simulink model "pattern_separation"  (R2019b)
settings: Solver=FixedStepAuto  StartTime=1  StopTime=simulationtime  FixedStep=stepsize  RelTol=1e-3
values from neighbouring files (symbols this model uses):
  a1 = 0.02    [simulation.m]
  a2 = 0.02    [simulation.m]
  b1 = 0.025    [simulation.m]
  b2 = 0.04    [simulation.m]
  c1 = -65    [simulation.m]
  C1 = normrnd(100,10,[1,nrofgranulecells])    [simulation.m]
  c2 = -65    [simulation.m]
  C2 = normrnd(100,10,[1,nrofinterneurons])    [simulation.m]
  d1 = 6    [simulation.m]
  d2 = 2    [simulation.m]
  inputset = inputsets{no_input}    [simulation.m]
  k1 = 0.25    [simulation.m]
  k2 = 0.25    [simulation.m]
  minimum_saturation_limit_1 = -80    [simulation.m]
  minimum_saturation_limit_2 = -100    [simulation.m]
  noumberofevents = 500    [simulation.m]
  Re = 230    [simulation.m]
  simulationtime = 2000    [simulation.m]
  stepsize = 1    [simulation.m]
  ve1 = -5    [simulation.m]
  ve2 = -80    [simulation.m]
  vr1 = -60    [simulation.m]
  vr2 = -65    [simulation.m]
  vt1 = -55    [simulation.m]
  vt2 = -48    [simulation.m]
undefined symbols (not defined in the file or in its folder): conductancemaxima1, conductancemaxima2, conductancemaxima3, decaytimes1, decaytimes2, decaytimes3, DiscIntNeverNeededParam, Nd, trace
(part 1 of 5)
settings Model: Creator=agorlewicz  LastModifiedBy=agorlewicz
settings OptimizationCC: BlockReduction=off  DefaultParameterBehavior=Inlined  BufferReuse=off

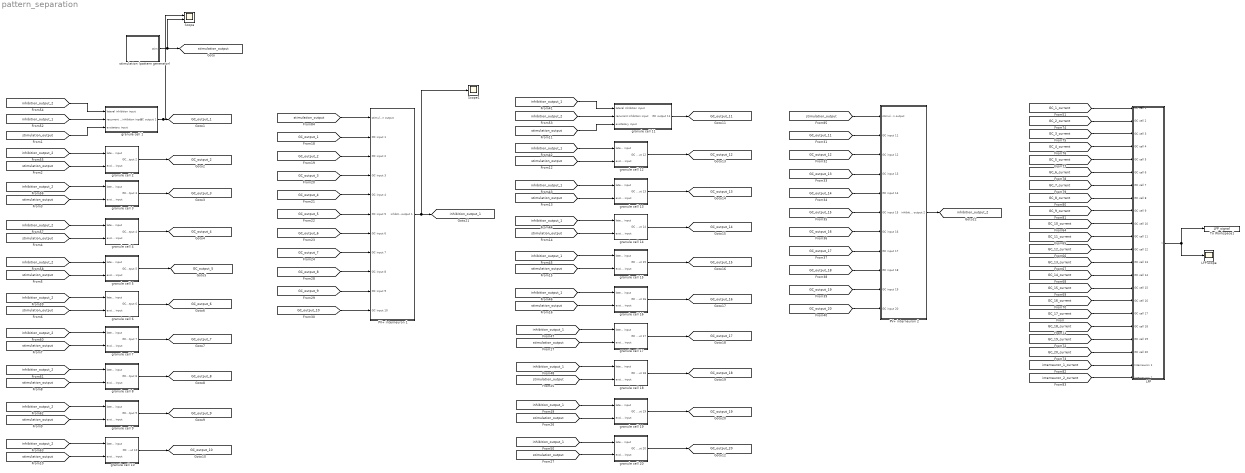
== system pattern_separation ==
  LFP : Subsystem
  LFP scope : Scope
  PV+ interneuron 1 : Subsystem
  PV+ interneuron 2 : Subsystem
  Scope : Scope  NumInputPorts=2
  Scope1 : Scope
  To Workspace1 : ToWorkspace  VariableName=LFP_signal  SampleTime=-1
  granule cell 1 : Subsystem
  granule cell 10 : Subsystem
  granule cell 11 : Subsystem
  granule cell 12 : Subsystem
  granule cell 13 : Subsystem
  granule cell 14 : Subsystem
  granule cell 15 : Subsystem
  granule cell 16 : Subsystem
  granule cell 17 : Subsystem
  granule cell 18 : Subsystem
  granule cell 19 : Subsystem
  granule cell 2 : Subsystem
  granule cell 20 : Subsystem
  granule cell 3 : Subsystem
  granule cell 4 : Subsystem
  granule cell 5 : Subsystem
  granule cell 6 : Subsystem
  granule cell 7 : Subsystem
  granule cell 8 : Subsystem
  granule cell 9 : Subsystem
  stimulation (pattern generator) : Subsystem
  tag scope: GC_output_10=global, GC_output_11=global, GC_output_12=global, GC_output_13=global, GC_output_14=global, GC_output_15=global, GC_output_16=global, GC_output_17=global, GC_output_18=global, GC_output_19=global, GC_output_1=global, GC_output_20=global, GC_output_2=global, GC_output_3=global, GC_output_4=global, GC_output_5=global, GC_output_6=global, GC_output_7=global, GC_output_8=global, GC_output_9=global, inhibition_output_1=global, inhibition_output_2=global, stimulation_output=global
  wires:
  stimulation (pattern generator)/1(stim) -> Scope/2, [stimulation_output]
  [stimulation_output] -> granule cell 1/3(excitatory input)
  [stimulation_output] -> granule cell 2/2(excitatory input)
  [stimulation_output] -> granule cell 3/2(excitatory input)
  [stimulation_output] -> granule cell 4/2(excitatory input)
  [stimulation_output] -> granule cell 5/2(excitatory input)
  [stimulation_output] -> granule cell 8/2(excitatory input)
  [stimulation_output] -> granule cell 7/2(excitatory input)
  [stimulation_output] -> granule cell 6/2(excitatory input)
  [stimulation_output] -> granule cell 9/2(excitatory input)
  [stimulation_output] -> granule cell 10/2(excitatory input)
  [stimulation_output] -> granule cell 11/3(excitatory input)
  [stimulation_output] -> granule cell 12/2(excitatory input)
  [stimulation_output] -> granule cell 13/2(excitatory input)
  [stimulation_output] -> granule cell 14/2(excitatory input)
  [stimulation_output] -> granule cell 15/2(excitatory input)
  [stimulation_output] -> granule cell 16/2(excitatory input)
  [stimulation_output] -> granule cell 18/2(excitatory input)
  [stimulation_output] -> granule cell 19/2(excitatory input)
  [stimulation_output] -> granule cell 17/2(excitatory input)
  [stimulation_output] -> granule cell 20/2(excitatory input)
  granule cell 1/1(GC output 1) -> Scope/1, [GC_output_1]
  [GC_output_1] -> PV+ interneuron 1/2(" GC input 1")
  granule cell 2/1(GC output 2) -> [GC_output_2]
  [GC_output_2] -> PV+ interneuron 1/3(" GC input 2")
  granule cell 3/1(GC output 3) -> [GC_output_3]
  [GC_output_3] -> PV+ interneuron 1/4(" GC input 3")
  granule cell 4/1(GC output 4) -> [GC_output_4]
  granule cell 5/1(GC output 5) -> [GC_output_5]
  granule cell 6/1(GC output 6) -> [GC_output_6]
  granule cell 7/1(GC output 7) -> [GC_output_7]
  granule cell 8/1(GC output 8) -> [GC_output_8]
  granule cell 9/1(GC output 9) -> [GC_output_9]
  granule cell 10/1(GC output 10) -> [GC_output_10]
  [GC_output_4] -> PV+ interneuron 1/5(" GC input 4")
  [GC_output_5] -> PV+ interneuron 1/6(" GC input 5")
  [GC_output_6] -> PV+ interneuron 1/7(" GC input 6")
  [GC_output_7] -> PV+ interneuron 1/8(" GC input 7")
  [GC_output_8] -> PV+ interneuron 1/9(" GC input 8")
  [GC_output_9] -> PV+ interneuron 1/10(GC input 9)
  [GC_output_10] -> PV+ interneuron 1/11(GC input 10)
  granule cell 11/1(GC output 11) -> [GC_output_11]
  granule cell 12/1(GC output 12) -> [GC_output_12]
  granule cell 13/1(GC output 13) -> [GC_output_13]
  granule cell 14/1(GC output 14) -> [GC_output_14]
  granule cell 15/1(GC output 15) -> [GC_output_15]
  granule cell 16/1(GC output 16) -> [GC_output_16]
  granule cell 17/1(GC output 17) -> [GC_output_17]
  granule cell 18/1(GC output 18) -> [GC_output_18]
  granule cell 19/1(GC output 19) -> [GC_output_19]
  granule cell 20/1(GC output 20) -> [GC_output_20]
  [GC_output_11] -> PV+ interneuron 2/2(" GC input 11")
  [GC_output_12] -> PV+ interneuron 2/3(" GC input 12")
  [GC_output_13] -> PV+ interneuron 2/4(" GC input 13")
  [GC_output_14] -> PV+ interneuron 2/5(" GC input 14")
  [GC_output_15] -> PV+ interneuron 2/6(" GC input 15")
  [GC_output_16] -> PV+ interneuron 2/7(" GC input 16")
  [GC_output_17] -> PV+ interneuron 2/8(" GC input 17")
  [GC_output_18] -> PV+ interneuron 2/9(" GC input 18")
  [GC_output_19] -> PV+ interneuron 2/10(GC input 19)
  [GC_output_20] -> PV+ interneuron 2/11(GC input 20)
  PV+ interneuron 1/1(inhibition output 1) -> [inhibition_output_1], Scope1/1
  [inhibition_output_1] -> granule cell 11/1(lateral inhibition input)
  [inhibition_output_1] -> granule cell 12/1(lateral inhibition input)
  [inhibition_output_1] -> granule cell 13/1(lateral inhibition input)
  [inhibition_output_1] -> granule cell 14/1(lateral inhibition input)
  [inhibition_output_1] -> granule cell 15/1(lateral inhibition input)
  [inhibition_output_1] -> granule cell 16/1(lateral inhibition input)
  [inhibition_output_1] -> granule cell 17/1(lateral inhibition input)
  [inhibition_output_1] -> granule cell 18/1(lateral inhibition input)
  [inhibition_output_1] -> granule cell 19/1(lateral inhibition input)
  [inhibition_output_1] -> granule cell 20/1(lateral inhibition input)
  [inhibition_output_1] -> granule cell 1/2(recurrent inhibition input)
  PV+ interneuron 2/1(inhibition output 2) -> [inhibition_output_2]
  [inhibition_output_2] -> granule cell 11/2(recurrent inhibition input)
  [inhibition_output_2] -> granule cell 1/1(lateral inhibition input)
  [inhibition_output_2] -> granule cell 2/1(lateral inhibition input)
  [inhibition_output_2] -> granule cell 3/1(lateral inhibition input)
  [inhibition_output_2] -> granule cell 4/1(lateral inhibition input)
  [inhibition_output_2] -> granule cell 5/1(lateral inhibition input)
  [inhibition_output_2] -> granule cell 6/1(lateral inhibition input)
  [inhibition_output_2] -> granule cell 7/1(lateral inhibition input)
  [inhibition_output_2] -> granule cell 8/1(lateral inhibition input)
  [inhibition_output_2] -> granule cell 9/1(lateral inhibition input)
  [inhibition_output_2] -> granule cell 10/1(lateral inhibition input)
  [GC_11_current] -> LFP/11(GC cell 11)
  [GC_9_current] -> LFP/9(GC cell 9)
  [GC_12_current] -> LFP/12(GC cell 12)
  [GC_14_current] -> LFP/14(GC cell 14)
  [GC_1_current] -> LFP/1("GC cell 1 ")
  [GC_13_current] -> LFP/13(GC cell 13)
  [GC_16_current] -> LFP/16(GC cell 16)
  [GC_17_current] -> LFP/17(GC cell 17)
  [GC_4_current] -> LFP/4("GC cell 4 ")
  [GC_5_current] -> LFP/5(GC cell 5)
  [GC_18_current] -> LFP/18(GC cell 18)
  [GC_8_current] -> LFP/8("GC cell 8 ")
  [GC_6_current] -> LFP/6(GC cell 6)
  [GC_7_current] -> LFP/7(GC cell 7)
  LFP/1(v) -> To Workspace1/1, LFP scope/1
  [GC_15_current] -> LFP/15(GC cell 15)
  [GC_3_current] -> LFP/3("GC cell 3 ")
  [GC_10_current] -> LFP/10(GC cell 10)
  [GC_19_current] -> LFP/19(GC cell 19)
  [GC_2_current] -> LFP/2("GC cell 2 ")
  [GC_20_current] -> LFP/20(GC cell 20)
  [interneuron_1_current] -> LFP/21(Interneuron 1)
  [interneuron_2_current] -> LFP/22(Interneuron 2)
  [stimulation_output] -> PV+ interneuron 1/1(stimulation output)
  [stimulation_output] -> PV+ interneuron 2/1(stimulation output)

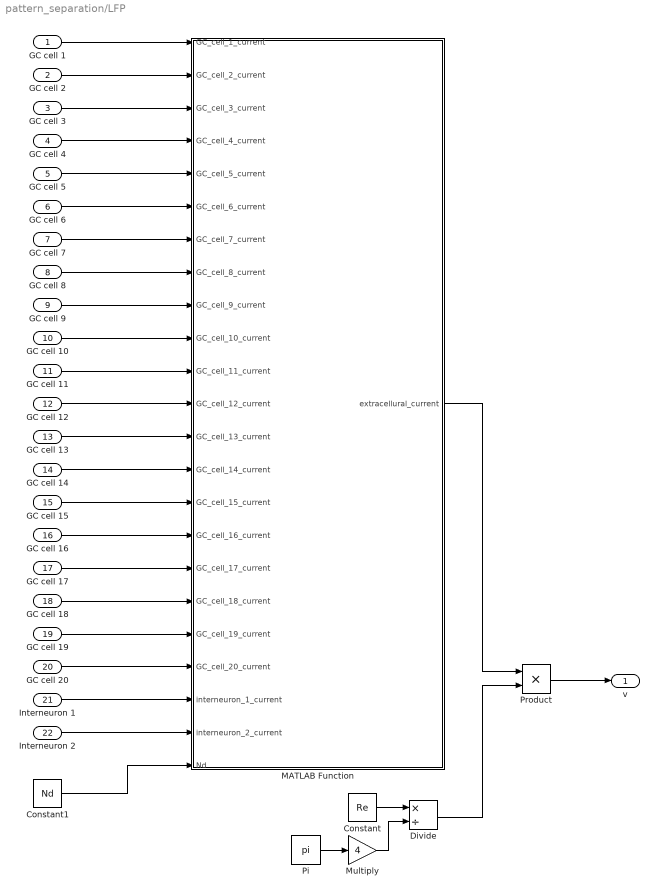
== system pattern_separation/LFP ==
  "GC cell 1 " : Inport
  "GC cell 2 " : Inport  Port=2
  "GC cell 3 " : Inport  Port=3
  "GC cell 4 " : Inport  Port=4
  GC cell 5 : Inport  Port=5
  GC cell 6 : Inport  Port=6
  GC cell 7 : Inport  Port=7
  "GC cell 8 " : Inport  Port=8
  GC cell 9 : Inport  Port=9
  GC cell 10 : Inport  Port=10
  GC cell 11 : Inport  Port=11
  GC cell 12 : Inport  Port=12
  GC cell 13 : Inport  Port=13
  GC cell 14 : Inport  Port=14
  GC cell 15 : Inport  Port=15
  GC cell 16 : Inport  Port=16
  GC cell 17 : Inport  Port=17
  GC cell 18 : Inport  Port=18
  GC cell 19 : Inport  Port=19
  GC cell 20 : Inport  Port=20
  Interneuron 1 : Inport  Port=21
  Interneuron 2 : Inport  Port=22
  Constant : Constant  Value=Re
  Constant1 : Constant  Value=Nd
  Divide : Product  Inputs=*/
  MATLAB Function : MATLAB Function  TreatAsAtomicUnit=on
  Multiply : Gain  Gain=4
  Pi : Constant  Value=pi  OutDataTypeStr=Inherit: Inherit via back propagation
  Product : Product
  v : Outport
  wires:
  Constant/1 -> Divide/1
  Pi/1 -> Multiply/1
  Multiply/1 -> Divide/2
  Constant1/1 -> MATLAB Function/23(Nd)
  MATLAB Function/1(extracellural_current) -> Product/1
  Divide/1 -> Product/2
  Product/1 -> v/1
  GC cell 20/1 -> MATLAB Function/20(GC_cell_20_current)
  GC cell 19/1 -> MATLAB Function/19(GC_cell_19_current)
  GC cell 18/1 -> MATLAB Function/18(GC_cell_18_current)
  GC cell 17/1 -> MATLAB Function/17(GC_cell_17_current)
  GC cell 16/1 -> MATLAB Function/16(GC_cell_16_current)
  GC cell 15/1 -> MATLAB Function/15(GC_cell_15_current)
  GC cell 14/1 -> MATLAB Function/14(GC_cell_14_current)
  GC cell 13/1 -> MATLAB Function/13(GC_cell_13_current)
  GC cell 12/1 -> MATLAB Function/12(GC_cell_12_current)
  GC cell 11/1 -> MATLAB Function/11(GC_cell_11_current)
  GC cell 10/1 -> MATLAB Function/10(GC_cell_10_current)
  GC cell 9/1 -> MATLAB Function/9(GC_cell_9_current)
  "GC cell 8 "/1 -> MATLAB Function/8(GC_cell_8_current)
  "GC cell 1 "/1 -> MATLAB Function/1(GC_cell_1_current)
  "GC cell 2 "/1 -> MATLAB Function/2(GC_cell_2_current)
  "GC cell 3 "/1 -> MATLAB Function/3(GC_cell_3_current)
  "GC cell 4 "/1 -> MATLAB Function/4(GC_cell_4_current)
  GC cell 5/1 -> MATLAB Function/5(GC_cell_5_current)
  GC cell 6/1 -> MATLAB Function/6(GC_cell_6_current)
  GC cell 7/1 -> MATLAB Function/7(GC_cell_7_current)
  Interneuron 1/1 -> MATLAB Function/21(interneuron_1_current)
  Interneuron 2/1 -> MATLAB Function/22(interneuron_2_current)

== system pattern_separation/PV+ interneuron 1 ==
  stimulation output : Inport
  " GC input 1" : Inport  Port=2
  " GC input 2" : Inport  Port=3
  " GC input 3" : Inport  Port=4
  " GC input 4" : Inport  Port=5
  " GC input 5" : Inport  Port=6
  " GC input 6" : Inport  Port=7
  " GC input 7" : Inport  Port=8
  " GC input 8" : Inport  Port=9
  GC input 9 : Inport  Port=10
  GC input 10 : Inport  Port=11
  Add2 : Sum  Inputs=+++++++++++
  Constant3 : Constant  SampleTime=-1
  Constant4 : Constant  Value=decaytimes3  SampleTime=-1
  Constant5 : Constant  Value=conductancemaxima3  SampleTime=-1
  Constant7 : Constant  Value=0  SampleTime=-1
  Data Type Conversion1 : DataTypeConversion  OutDataTypeStr=double
  Discrete-Time Integrator1 : DiscreteIntegrator  gainval=1/stepsize  ExternalReset=sampled level  SampleTime=-1  ICPrevOutput=DiscIntNeverNeededParam  ICPrevScaledInput=DiscIntNeverNeededParam
  Floor1 : Rounding
  Integrator1 : Integrator  ExternalReset=level hold
  MATLAB Function1 : MATLAB Function  TreatAsAtomicUnit=on
  Memory1 : Memory  InheritSampleTime=on
  Product2 : Product
  Relational Operator1 : RelationalOperator  Operator=>  OutDataTypeStr=boolean  RndMeth=Simplest
  Uniform Random Number1 : UniformRandomNumber  Minimum=1  Maximum=noumberofevents  Seed=41  SampleTime=stepsize
  interneuron : Subsystem
  single exp EPSCs generator (ff synapse) : Subsystem
  inhibition output 1 : Outport
  tag scope: interneuron_1_current=global
  wires:
  interneuron/1(output) -> inhibition output 1/1
  Memory1/1 -> Product2/1, Discrete-Time Integrator1/2, Integrator1/2
  Uniform Random Number1/1 -> Floor1/1
  Constant4/1 -> MATLAB Function1/2(decaytimes3)
  Floor1/1 -> Product2/2
  Constant5/1 -> MATLAB Function1/3(conductancemaxima3)
  Integrator1/1 -> single exp EPSCs generator (ff synapse)/1(event time)
  MATLAB Function1/1(decaytime) -> single exp EPSCs generator (ff synapse)/2(decay time constant)
  MATLAB Function1/2(conductancemaximum) -> single exp EPSCs generator (ff synapse)/3(conductance maximum)
  Constant3/1 -> Integrator1/1
  Product2/1 -> Discrete-Time Integrator1/1
  Discrete-Time Integrator1/1 -> MATLAB Function1/1(eventnoumber)
  single exp EPSCs generator (ff synapse)/1(postsynaptic current) -> [interneuron_1_current], interneuron/1(postsynaptic current)
  Constant7/1 -> Relational Operator1/2
  Relational Operator1/1 -> Data Type Conversion1/1
  " GC input 1"/1 -> Add2/2
  " GC input 2"/1 -> Add2/3
  Add2/1 -> Relational Operator1/1
  Data Type Conversion1/1 -> Memory1/1
  " GC input 3"/1 -> Add2/4
  " GC input 4"/1 -> Add2/5
  " GC input 5"/1 -> Add2/6
  " GC input 6"/1 -> Add2/7
  " GC input 7"/1 -> Add2/8
  " GC input 8"/1 -> Add2/9
  GC input 9/1 -> Add2/10
  GC input 10/1 -> Add2/11
  stimulation output/1 -> Add2/1

== system pattern_separation/PV+ interneuron 2 ==
  stimulation output : Inport
  " GC input 11" : Inport  Port=2
  " GC input 12" : Inport  Port=3
  " GC input 13" : Inport  Port=4
  " GC input 14" : Inport  Port=5
  " GC input 15" : Inport  Port=6
  " GC input 16" : Inport  Port=7
  " GC input 17" : Inport  Port=8
  " GC input 18" : Inport  Port=9
  GC input 19 : Inport  Port=10
  GC input 20 : Inport  Port=11
  Add2 : Sum  Inputs=+++++++++++
  Constant3 : Constant  SampleTime=-1
  Constant4 : Constant  Value=decaytimes3  SampleTime=-1
  Constant5 : Constant  Value=conductancemaxima3  SampleTime=-1
  Constant7 : Constant  Value=0  SampleTime=-1
  Data Type Conversion1 : DataTypeConversion  OutDataTypeStr=double
  Discrete-Time Integrator1 : DiscreteIntegrator  gainval=1/stepsize  ExternalReset=sampled level  SampleTime=-1  ICPrevOutput=DiscIntNeverNeededParam  ICPrevScaledInput=DiscIntNeverNeededParam
  Floor1 : Rounding
  Integrator1 : Integrator  ExternalReset=level hold
  MATLAB Function1 : MATLAB Function  TreatAsAtomicUnit=on
  Memory1 : Memory  InheritSampleTime=on
  Product2 : Product
  Relational Operator1 : RelationalOperator  Operator=>  OutDataTypeStr=boolean  RndMeth=Simplest
  Uniform Random Number1 : UniformRandomNumber  Minimum=1  Maximum=noumberofevents  Seed=42  SampleTime=stepsize
  interneuron : Subsystem
  single exp EPSCs generator (ff synapse) : Subsystem
  inhibition output 2 : Outport
  tag scope: interneuron_2_current=global
  wires:
  interneuron/1(output) -> inhibition output 2/1
  Memory1/1 -> Product2/1, Discrete-Time Integrator1/2, Integrator1/2
  Uniform Random Number1/1 -> Floor1/1
  Constant4/1 -> MATLAB Function1/2(decaytimes3)
  Floor1/1 -> Product2/2
  Constant5/1 -> MATLAB Function1/3(conductancemaxima3)
  Integrator1/1 -> single exp EPSCs generator (ff synapse)/1(event time)
  MATLAB Function1/1(decaytime) -> single exp EPSCs generator (ff synapse)/2(decay time constant)
  MATLAB Function1/2(conductancemaximum) -> single exp EPSCs generator (ff synapse)/3(conductance maximum)
  Constant3/1 -> Integrator1/1
  Product2/1 -> Discrete-Time Integrator1/1
  Discrete-Time Integrator1/1 -> MATLAB Function1/1(eventnoumber)
  single exp EPSCs generator (ff synapse)/1(postsynaptic current) -> [interneuron_2_current], interneuron/1(postsynaptic current)
  Constant7/1 -> Relational Operator1/2
  Relational Operator1/1 -> Data Type Conversion1/1
  " GC input 11"/1 -> Add2/2
  " GC input 12"/1 -> Add2/3
  Add2/1 -> Relational Operator1/1
  Data Type Conversion1/1 -> Memory1/1
  " GC input 13"/1 -> Add2/4
  " GC input 14"/1 -> Add2/5
  " GC input 15"/1 -> Add2/6
  " GC input 16"/1 -> Add2/7
  " GC input 17"/1 -> Add2/8
  " GC input 18"/1 -> Add2/9
  GC input 19/1 -> Add2/10
  GC input 20/1 -> Add2/11
  stimulation output/1 -> Add2/1

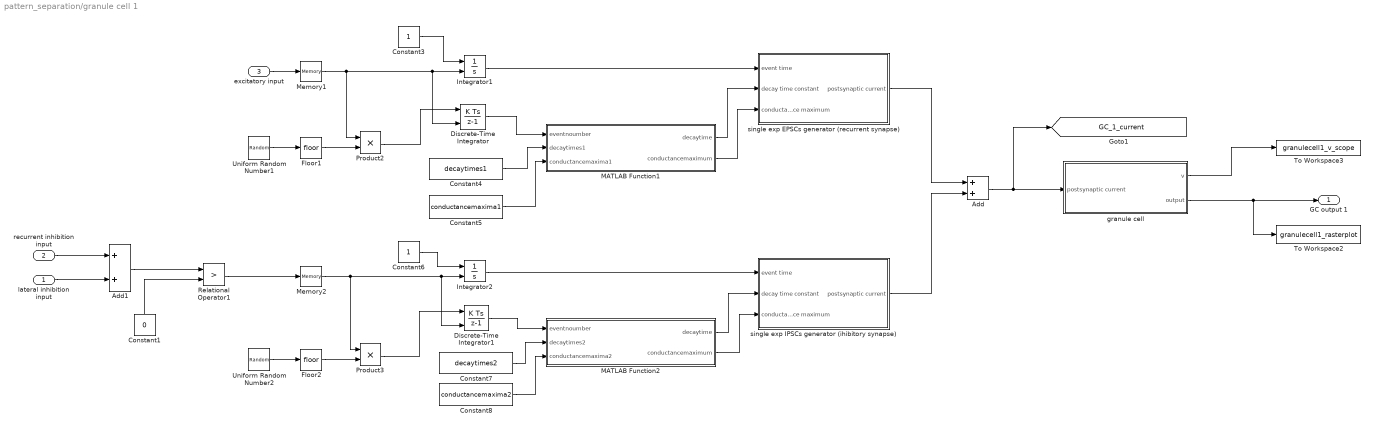
== system pattern_separation/granule cell 1 ==
  lateral inhibition input : Inport
  recurrent inhibition input : Inport  Port=2
  excitatory input : Inport  Port=3
  Add : Sum
  Add1 : Sum
  Constant1 : Constant  Value=0  SampleTime=-1
  Constant3 : Constant  SampleTime=-1
  Constant4 : Constant  Value=decaytimes1  SampleTime=-1
  Constant5 : Constant  Value=conductancemaxima1  SampleTime=-1
  Constant6 : Constant  SampleTime=-1
  Constant7 : Constant  Value=decaytimes2  SampleTime=-1
  Constant8 : Constant  Value=conductancemaxima2  SampleTime=-1
  Discrete-Time Integrator : DiscreteIntegrator  gainval=1/stepsize  ExternalReset=sampled level  SampleTime=-1  ICPrevOutput=DiscIntNeverNeededParam  ICPrevScaledInput=DiscIntNeverNeededParam
  Discrete-Time Integrator1 : DiscreteIntegrator  gainval=1/stepsize  ExternalReset=sampled level  SampleTime=-1  ICPrevOutput=DiscIntNeverNeededParam  ICPrevScaledInput=DiscIntNeverNeededParam
  Floor1 : Rounding
  Floor2 : Rounding
  Integrator1 : Integrator  ExternalReset=level hold
  Integrator2 : Integrator  ExternalReset=level hold
  MATLAB Function1 : MATLAB Function  TreatAsAtomicUnit=on
  MATLAB Function2 : MATLAB Function  TreatAsAtomicUnit=on
  Memory1 : Memory  InheritSampleTime=on
  Memory2 : Memory  InheritSampleTime=on
  Product2 : Product
  Product3 : Product
  Relational Operator1 : RelationalOperator  Operator=>  OutDataTypeStr=boolean  RndMeth=Simplest
  To Workspace2 : ToWorkspace  VariableName=granulecell1_rasterplot  SampleTime=-1
  To Workspace3 : ToWorkspace  VariableName=granulecell1_v_scope  SampleTime=-1
  Uniform Random Number1 : UniformRandomNumber  Minimum=1  Maximum=noumberofevents  Seed=1  SampleTime=stepsize
  Uniform Random Number2 : UniformRandomNumber  Minimum=1  Maximum=noumberofevents  Seed=2  SampleTime=stepsize
  granule cell : Subsystem
  single exp EPSCs generator (recurrent synapse) : Subsystem
  single exp IPSCs generator (ihibitory synapse) : Subsystem
  GC output 1 : Outport
  tag scope: GC_1_current=global
  wires:
  Discrete-Time Integrator/1 -> MATLAB Function1/1(eventnoumber)
  Memory1/1 -> Product2/1, Discrete-Time Integrator/2, Integrator1/2
  granule cell/2(output) -> To Workspace2/1, GC output 1/1
  MATLAB Function2/2(conductancemaximum) -> single exp IPSCs generator (ihibitory synapse)/3(conductance maximum)
  Uniform Random Number1/1 -> Floor1/1
  Uniform Random Number2/1 -> Floor2/1
  excitatory input/1 -> Memory1/1
  single exp EPSCs generator (recurrent synapse)/1(postsynaptic current) -> Add/1
  Product3/1 -> Discrete-Time Integrator1/1
  Floor1/1 -> Product2/2
  Constant3/1 -> Integrator1/1
  single exp IPSCs generator (ihibitory synapse)/1(postsynaptic current) -> Add/2
  Product2/1 -> Discrete-Time Integrator/1
  granule cell/1(v) -> To Workspace3/1
  MATLAB Function1/1(decaytime) -> single exp EPSCs generator (recurrent synapse)/2(decay time constant)
  MATLAB Function2/1(decaytime) -> single exp IPSCs generator (ihibitory synapse)/2(decay time constant)
  Integrator1/1 -> single exp EPSCs generator (recurrent synapse)/1(event time)
  Constant5/1 -> MATLAB Function1/3(conductancemaxima1)
  Memory2/1 -> Product3/1, Discrete-Time Integrator1/2, Integrator2/2
  MATLAB Function1/2(conductancemaximum) -> single exp EPSCs generator (recurrent synapse)/3(conductance maximum)
  Constant6/1 -> Integrator2/1
  Constant4/1 -> MATLAB Function1/2(decaytimes1)
  Constant7/1 -> MATLAB Function2/2(decaytimes2)
  Constant8/1 -> MATLAB Function2/3(conductancemaxima2)
  Floor2/1 -> Product3/2
  Integrator2/1 -> single exp IPSCs generator (ihibitory synapse)/1(event time)
  Discrete-Time Integrator1/1 -> MATLAB Function2/1(eventnoumber)
  Add1/1 -> Relational Operator1/1
  Constant1/1 -> Relational Operator1/2
  recurrent inhibition input/1 -> Add1/1
  lateral inhibition input/1 -> Add1/2
  Relational Operator1/1 -> Memory2/1
  Add/1 -> granule cell/1(postsynaptic current), [GC_1_current]

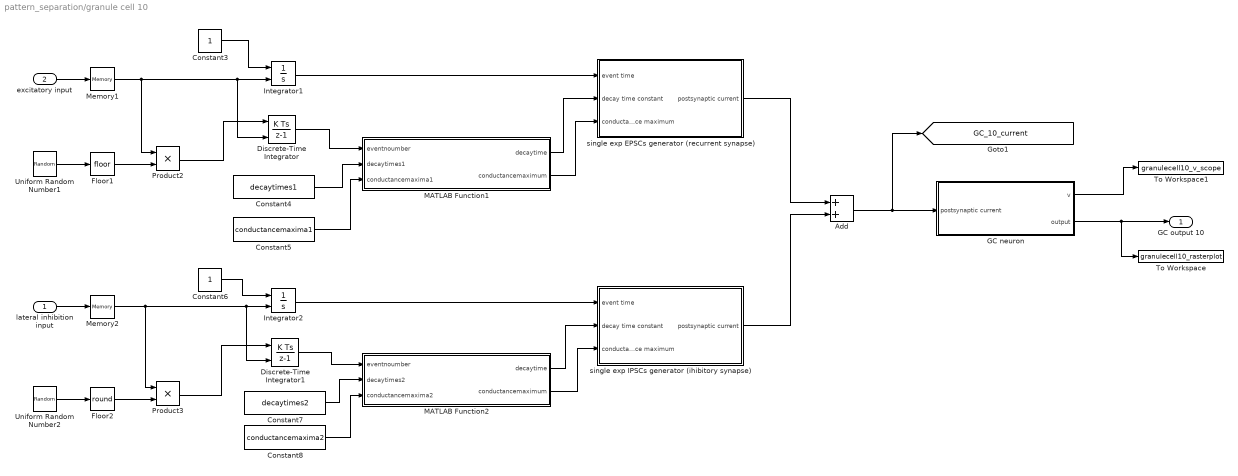
== system pattern_separation/granule cell 10 ==
  lateral inhibition input : Inport
  excitatory input : Inport  Port=2
  Add : Sum
  Constant3 : Constant  SampleTime=-1
  Constant4 : Constant  Value=decaytimes1  SampleTime=-1
  Constant5 : Constant  Value=conductancemaxima1  SampleTime=-1
  Constant6 : Constant  SampleTime=-1
  Constant7 : Constant  Value=decaytimes2  SampleTime=-1
  Constant8 : Constant  Value=conductancemaxima2  VectorParams1D=off  SampleTime=-1
  Discrete-Time Integrator : DiscreteIntegrator  gainval=1/stepsize  ExternalReset=sampled level  SampleTime=-1  ICPrevOutput=DiscIntNeverNeededParam  ICPrevScaledInput=DiscIntNeverNeededParam
  Discrete-Time Integrator1 : DiscreteIntegrator  gainval=1/stepsize  ExternalReset=sampled level  SampleTime=-1  ICPrevOutput=DiscIntNeverNeededParam  ICPrevScaledInput=DiscIntNeverNeededParam
  Floor1 : Rounding
  Floor2 : Rounding  Operator=round
  GC neuron : Subsystem
  Integrator1 : Integrator  ExternalReset=level hold
  Integrator2 : Integrator  ExternalReset=level hold
  MATLAB Function1 : MATLAB Function  TreatAsAtomicUnit=on
  MATLAB Function2 : MATLAB Function  TreatAsAtomicUnit=on
  Memory1 : Memory  InheritSampleTime=on
  Memory2 : Memory  InheritSampleTime=on
  Product2 : Product
  Product3 : Product
  To Workspace : ToWorkspace  VariableName=granulecell10_rasterplot  SampleTime=-1
  To Workspace1 : ToWorkspace  VariableName=granulecell10_v_scope  SampleTime=-1
  Uniform Random Number1 : UniformRandomNumber  Minimum=1  Maximum=noumberofevents  Seed=19  SampleTime=stepsize
  Uniform Random Number2 : UniformRandomNumber  Minimum=1  Maximum=noumberofevents  Seed=20  SampleTime=stepsize
  single exp EPSCs generator (recurrent synapse) : Subsystem
  single exp IPSCs generator (ihibitory synapse) : Subsystem
  GC output 10 : Outport
  tag scope: GC_10_current=global
  wires:
  GC neuron/1(v) -> To Workspace1/1
  GC neuron/2(output) -> To Workspace/1, GC output 10/1
  Constant7/1 -> MATLAB Function2/2(decaytimes2)
  Constant8/1 -> MATLAB Function2/3(conductancemaxima2)
  Discrete-Time Integrator1/1 -> MATLAB Function2/1(eventnoumber)
  Floor2/1 -> Product3/2
  Discrete-Time Integrator/1 -> MATLAB Function1/1(eventnoumber)
  MATLAB Function2/1(decaytime) -> single exp IPSCs generator (ihibitory synapse)/2(decay time constant)
  Product2/1 -> Discrete-Time Integrator/1
  Integrator2/1 -> single exp IPSCs generator (ihibitory synapse)/1(event time)
  Add/1 -> [GC_10_current], GC neuron/1(postsynaptic current)
  Memory2/1 -> Product3/1, Discrete-Time Integrator1/2, Integrator2/2
  single exp IPSCs generator (ihibitory synapse)/1(postsynaptic current) -> Add/2
  MATLAB Function1/1(decaytime) -> single exp EPSCs generator (recurrent synapse)/2(decay time constant)
  MATLAB Function1/2(conductancemaximum) -> single exp EPSCs generator (recurrent synapse)/3(conductance maximum)
  Constant6/1 -> Integrator2/1
  Constant4/1 -> MATLAB Function1/2(decaytimes1)
  Constant5/1 -> MATLAB Function1/3(conductancemaxima1)
  Integrator1/1 -> single exp EPSCs generator (recurrent synapse)/1(event time)
  Product3/1 -> Discrete-Time Integrator1/1
  single exp EPSCs generator (recurrent synapse)/1(postsynaptic current) -> Add/1
  lateral inhibition input/1 -> Memory2/1
  Floor1/1 -> Product2/2
  MATLAB Function2/2(conductancemaximum) -> single exp IPSCs generator (ihibitory synapse)/3(conductance maximum)
  Memory1/1 -> Product2/1, Discrete-Time Integrator/2, Integrator1/2
  Uniform Random Number1/1 -> Floor1/1
  Constant3/1 -> Integrator1/1
  Uniform Random Number2/1 -> Floor2/1
  excitatory input/1 -> Memory1/1

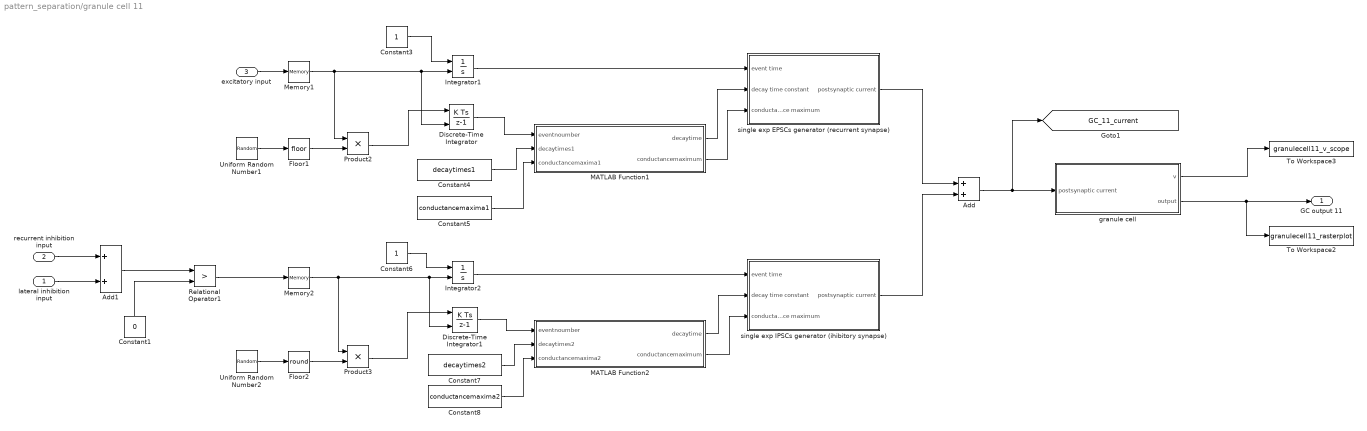
== system pattern_separation/granule cell 11 ==
  lateral inhibition input : Inport
  recurrent inhibition input : Inport  Port=2
  excitatory input : Inport  Port=3
  Add : Sum
  Add1 : Sum
  Constant1 : Constant  Value=0  SampleTime=-1
  Constant3 : Constant  SampleTime=-1
  Constant4 : Constant  Value=decaytimes1  SampleTime=-1
  Constant5 : Constant  Value=conductancemaxima1  SampleTime=-1
  Constant6 : Constant  SampleTime=-1
  Constant7 : Constant  Value=decaytimes2  SampleTime=-1
  Constant8 : Constant  Value=conductancemaxima2  SampleTime=-1
  Discrete-Time Integrator : DiscreteIntegrator  gainval=1/stepsize  ExternalReset=sampled level  SampleTime=-1  ICPrevOutput=DiscIntNeverNeededParam  ICPrevScaledInput=DiscIntNeverNeededParam
  Discrete-Time Integrator1 : DiscreteIntegrator  gainval=1/stepsize  ExternalReset=sampled level  SampleTime=-1  ICPrevOutput=DiscIntNeverNeededParam  ICPrevScaledInput=DiscIntNeverNeededParam
  Floor1 : Rounding
  Floor2 : Rounding  Operator=round
  Integrator1 : Integrator  ExternalReset=level hold
  Integrator2 : Integrator  ExternalReset=level hold
  MATLAB Function1 : MATLAB Function  TreatAsAtomicUnit=on
  MATLAB Function2 : MATLAB Function  TreatAsAtomicUnit=on
  Memory1 : Memory  InheritSampleTime=on
  Memory2 : Memory  InheritSampleTime=on
  Product2 : Product
  Product3 : Product
  Relational Operator1 : RelationalOperator  Operator=>  OutDataTypeStr=boolean  RndMeth=Simplest
  To Workspace2 : ToWorkspace  VariableName=granulecell11_rasterplot  SampleTime=-1
  To Workspace3 : ToWorkspace  VariableName=granulecell11_v_scope  SampleTime=-1
  Uniform Random Number1 : UniformRandomNumber  Minimum=1  Maximum=noumberofevents  Seed=21  SampleTime=stepsize
  Uniform Random Number2 : UniformRandomNumber  Minimum=1  Maximum=noumberofevents  Seed=22  SampleTime=stepsize
  granule cell : Subsystem
  single exp EPSCs generator (recurrent synapse) : Subsystem
  single exp IPSCs generator (ihibitory synapse) : Subsystem
  GC output 11 : Outport
  tag scope: GC_11_current=global
  wires:
  Discrete-Time Integrator/1 -> MATLAB Function1/1(eventnoumber)
  Memory1/1 -> Product2/1, Discrete-Time Integrator/2, Integrator1/2
  granule cell/2(output) -> GC output 11/1, To Workspace2/1
  MATLAB Function2/2(conductancemaximum) -> single exp IPSCs generator (ihibitory synapse)/3(conductance maximum)
  Uniform Random Number1/1 -> Floor1/1
  Uniform Random Number2/1 -> Floor2/1
  excitatory input/1 -> Memory1/1
  single exp EPSCs generator (recurrent synapse)/1(postsynaptic current) -> Add/1
  Product3/1 -> Discrete-Time Integrator1/1
  Floor1/1 -> Product2/2
  Constant3/1 -> Integrator1/1
  single exp IPSCs generator (ihibitory synapse)/1(postsynaptic current) -> Add/2
  Product2/1 -> Discrete-Time Integrator/1
  granule cell/1(v) -> To Workspace3/1
  MATLAB Function1/1(decaytime) -> single exp EPSCs generator (recurrent synapse)/2(decay time constant)
  MATLAB Function2/1(decaytime) -> single exp IPSCs generator (ihibitory synapse)/2(decay time constant)
  Add/1 -> [GC_11_current], granule cell/1(postsynaptic current)
  Integrator1/1 -> single exp EPSCs generator (recurrent synapse)/1(event time)
  Constant5/1 -> MATLAB Function1/3(conductancemaxima1)
  Memory2/1 -> Product3/1, Discrete-Time Integrator1/2, Integrator2/2
  MATLAB Function1/2(conductancemaximum) -> single exp EPSCs generator (recurrent synapse)/3(conductance maximum)
  Constant6/1 -> Integrator2/1
  Constant4/1 -> MATLAB Function1/2(decaytimes1)
  Constant7/1 -> MATLAB Function2/2(decaytimes2)
  Constant8/1 -> MATLAB Function2/3(conductancemaxima2)
  Floor2/1 -> Product3/2
  Integrator2/1 -> single exp IPSCs generator (ihibitory synapse)/1(event time)
  Discrete-Time Integrator1/1 -> MATLAB Function2/1(eventnoumber)
  Relational Operator1/1 -> Memory2/1
  Add1/1 -> Relational Operator1/1
  Constant1/1 -> Relational Operator1/2
  lateral inhibition input/1 -> Add1/2
  recurrent inhibition input/1 -> Add1/1

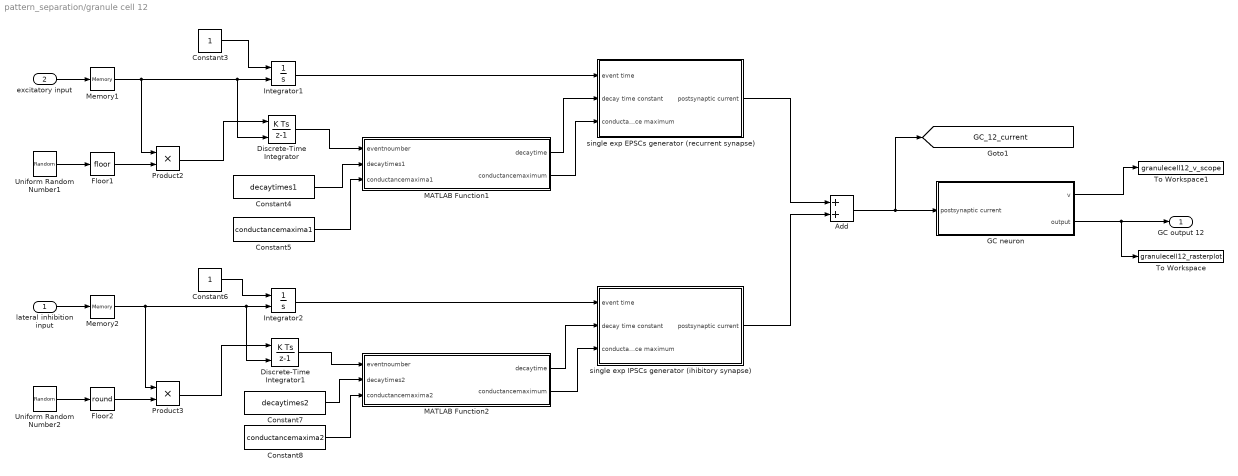
== system pattern_separation/granule cell 12 ==
  lateral inhibition input : Inport
  excitatory input : Inport  Port=2
  Add : Sum
  Constant3 : Constant  SampleTime=-1
  Constant4 : Constant  Value=decaytimes1  SampleTime=-1
  Constant5 : Constant  Value=conductancemaxima1  SampleTime=-1
  Constant6 : Constant  SampleTime=-1
  Constant7 : Constant  Value=decaytimes2  SampleTime=-1
  Constant8 : Constant  Value=conductancemaxima2  VectorParams1D=off  SampleTime=-1
  Discrete-Time Integrator : DiscreteIntegrator  gainval=1/stepsize  ExternalReset=sampled level  SampleTime=-1  ICPrevOutput=DiscIntNeverNeededParam  ICPrevScaledInput=DiscIntNeverNeededParam
  Discrete-Time Integrator1 : DiscreteIntegrator  gainval=1/stepsize  ExternalReset=sampled level  SampleTime=-1  ICPrevOutput=DiscIntNeverNeededParam  ICPrevScaledInput=DiscIntNeverNeededParam
  Floor1 : Rounding
  Floor2 : Rounding  Operator=round
  GC neuron : Subsystem
  Integrator1 : Integrator  ExternalReset=level hold
  Integrator2 : Integrator  ExternalReset=level hold
  MATLAB Function1 : MATLAB Function  TreatAsAtomicUnit=on
  MATLAB Function2 : MATLAB Function  TreatAsAtomicUnit=on
  Memory1 : Memory  InheritSampleTime=on
  Memory2 : Memory  InheritSampleTime=on
  Product2 : Product
  Product3 : Product
  To Workspace : ToWorkspace  VariableName=granulecell12_rasterplot  SampleTime=-1
  To Workspace1 : ToWorkspace  VariableName=granulecell12_v_scope  SampleTime=-1
  Uniform Random Number1 : UniformRandomNumber  Minimum=1  Maximum=noumberofevents  Seed=23  SampleTime=stepsize
  Uniform Random Number2 : UniformRandomNumber  Minimum=1  Maximum=noumberofevents  Seed=24  SampleTime=stepsize
  single exp EPSCs generator (recurrent synapse) : Subsystem
  single exp IPSCs generator (ihibitory synapse) : Subsystem
  GC output 12 : Outport
  tag scope: GC_12_current=global
  wires:
  GC neuron/1(v) -> To Workspace1/1
  GC neuron/2(output) -> To Workspace/1, GC output 12/1
  Constant7/1 -> MATLAB Function2/2(decaytimes2)
  Constant8/1 -> MATLAB Function2/3(conductancemaxima2)
  Discrete-Time Integrator1/1 -> MATLAB Function2/1(eventnoumber)
  Floor2/1 -> Product3/2
  Discrete-Time Integrator/1 -> MATLAB Function1/1(eventnoumber)
  MATLAB Function2/1(decaytime) -> single exp IPSCs generator (ihibitory synapse)/2(decay time constant)
  Product2/1 -> Discrete-Time Integrator/1
  Integrator2/1 -> single exp IPSCs generator (ihibitory synapse)/1(event time)
  Add/1 -> [GC_12_current], GC neuron/1(postsynaptic current)
  Memory2/1 -> Product3/1, Discrete-Time Integrator1/2, Integrator2/2
  single exp IPSCs generator (ihibitory synapse)/1(postsynaptic current) -> Add/2
  MATLAB Function1/1(decaytime) -> single exp EPSCs generator (recurrent synapse)/2(decay time constant)
  MATLAB Function1/2(conductancemaximum) -> single exp EPSCs generator (recurrent synapse)/3(conductance maximum)
  Constant6/1 -> Integrator2/1
  Constant4/1 -> MATLAB Function1/2(decaytimes1)
  Constant5/1 -> MATLAB Function1/3(conductancemaxima1)
  Integrator1/1 -> single exp EPSCs generator (recurrent synapse)/1(event time)
  Product3/1 -> Discrete-Time Integrator1/1
  single exp EPSCs generator (recurrent synapse)/1(postsynaptic current) -> Add/1
  lateral inhibition input/1 -> Memory2/1
  Floor1/1 -> Product2/2
  MATLAB Function2/2(conductancemaximum) -> single exp IPSCs generator (ihibitory synapse)/3(conductance maximum)
  Memory1/1 -> Product2/1, Discrete-Time Integrator/2, Integrator1/2
  Uniform Random Number1/1 -> Floor1/1
  Constant3/1 -> Integrator1/1
  Uniform Random Number2/1 -> Floor2/1
  excitatory input/1 -> Memory1/1

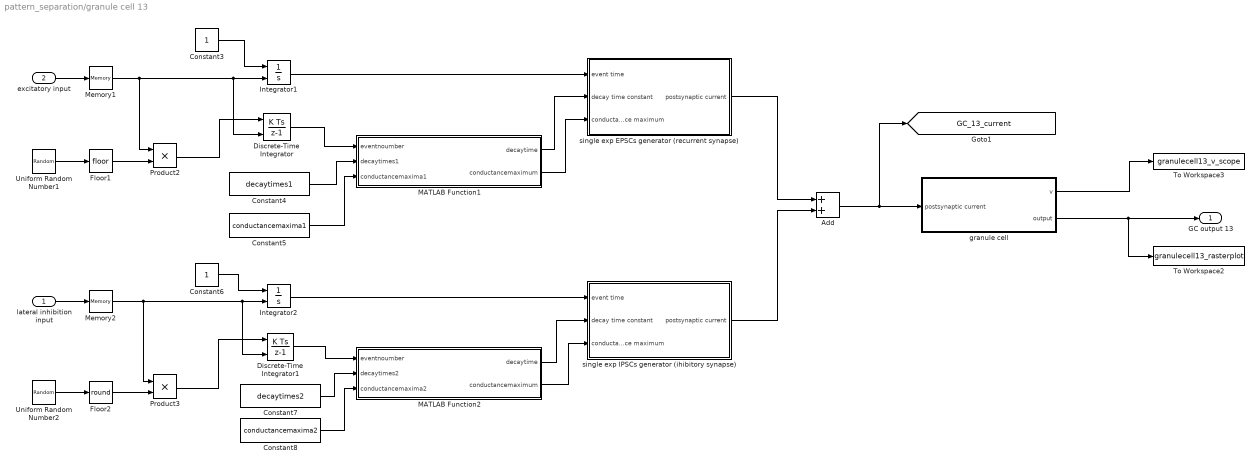
== system pattern_separation/granule cell 13 ==
  lateral inhibition input : Inport
  excitatory input : Inport  Port=2
  Add : Sum
  Constant3 : Constant  SampleTime=-1
  Constant4 : Constant  Value=decaytimes1  SampleTime=-1
  Constant5 : Constant  Value=conductancemaxima1  SampleTime=-1
  Constant6 : Constant  SampleTime=-1
  Constant7 : Constant  Value=decaytimes2  SampleTime=-1
  Constant8 : Constant  Value=conductancemaxima2  SampleTime=-1
  Discrete-Time Integrator : DiscreteIntegrator  gainval=1/stepsize  ExternalReset=sampled level  SampleTime=-1  ICPrevOutput=DiscIntNeverNeededParam  ICPrevScaledInput=DiscIntNeverNeededParam
  Discrete-Time Integrator1 : DiscreteIntegrator  gainval=1/stepsize  ExternalReset=sampled level  SampleTime=-1  ICPrevOutput=DiscIntNeverNeededParam  ICPrevScaledInput=DiscIntNeverNeededParam
  Floor1 : Rounding
  Floor2 : Rounding  Operator=round
  Integrator1 : Integrator  ExternalReset=level hold
  Integrator2 : Integrator  ExternalReset=level hold
  MATLAB Function1 : MATLAB Function  TreatAsAtomicUnit=on
  MATLAB Function2 : MATLAB Function  TreatAsAtomicUnit=on
  Memory1 : Memory  InheritSampleTime=on
  Memory2 : Memory  InheritSampleTime=on
  Product2 : Product
  Product3 : Product
  To Workspace2 : ToWorkspace  VariableName=granulecell13_rasterplot  SampleTime=-1
  To Workspace3 : ToWorkspace  VariableName=granulecell13_v_scope  SampleTime=-1
  Uniform Random Number1 : UniformRandomNumber  Minimum=1  Maximum=noumberofevents  Seed=25  SampleTime=stepsize
  Uniform Random Number2 : UniformRandomNumber  Minimum=1  Maximum=noumberofevents  Seed=26  SampleTime=stepsize
  granule cell : Subsystem
  single exp EPSCs generator (recurrent synapse) : Subsystem
  single exp IPSCs generator (ihibitory synapse) : Subsystem
  GC output 13 : Outport
  tag scope: GC_13_current=global
  wires:
  Discrete-Time Integrator/1 -> MATLAB Function1/1(eventnoumber)
  Memory1/1 -> Product2/1, Discrete-Time Integrator/2, Integrator1/2
  granule cell/2(output) -> GC output 13/1, To Workspace2/1
  MATLAB Function2/2(conductancemaximum) -> single exp IPSCs generator (ihibitory synapse)/3(conductance maximum)
  lateral inhibition input/1 -> Memory2/1
  Uniform Random Number1/1 -> Floor1/1
  Uniform Random Number2/1 -> Floor2/1
  excitatory input/1 -> Memory1/1
  single exp EPSCs generator (recurrent synapse)/1(postsynaptic current) -> Add/1
  Product3/1 -> Discrete-Time Integrator1/1
  Floor1/1 -> Product2/2
  Constant3/1 -> Integrator1/1
  single exp IPSCs generator (ihibitory synapse)/1(postsynaptic current) -> Add/2
  Product2/1 -> Discrete-Time Integrator/1
  granule cell/1(v) -> To Workspace3/1
  MATLAB Function1/1(decaytime) -> single exp EPSCs generator (recurrent synapse)/2(decay time constant)
  MATLAB Function2/1(decaytime) -> single exp IPSCs generator (ihibitory synapse)/2(decay time constant)
  Add/1 -> [GC_13_current], granule cell/1(postsynaptic current)
  Integrator1/1 -> single exp EPSCs generator (recurrent synapse)/1(event time)
  Constant5/1 -> MATLAB Function1/3(conductancemaxima1)
  Memory2/1 -> Product3/1, Discrete-Time Integrator1/2, Integrator2/2
  MATLAB Function1/2(conductancemaximum) -> single exp EPSCs generator (recurrent synapse)/3(conductance maximum)
  Constant6/1 -> Integrator2/1
  Constant4/1 -> MATLAB Function1/2(decaytimes1)
  Constant7/1 -> MATLAB Function2/2(decaytimes2)
  Constant8/1 -> MATLAB Function2/3(conductancemaxima2)
  Floor2/1 -> Product3/2
  Integrator2/1 -> single exp IPSCs generator (ihibitory synapse)/1(event time)
  Discrete-Time Integrator1/1 -> MATLAB Function2/1(eventnoumber)

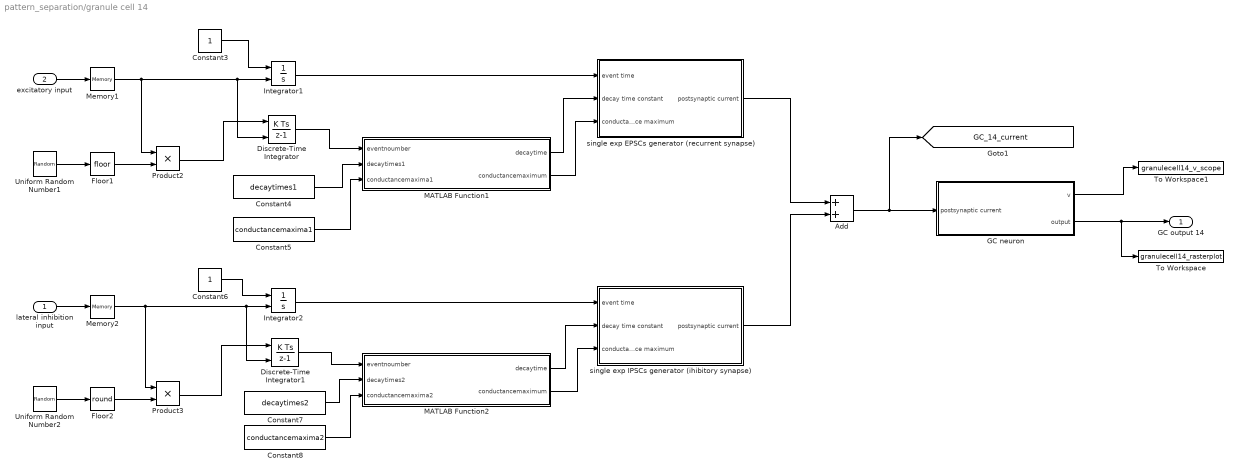
== system pattern_separation/granule cell 14 ==
  lateral inhibition input : Inport
  excitatory input : Inport  Port=2
  Add : Sum
  Constant3 : Constant  SampleTime=-1
  Constant4 : Constant  Value=decaytimes1  SampleTime=-1
  Constant5 : Constant  Value=conductancemaxima1  SampleTime=-1
  Constant6 : Constant  SampleTime=-1
  Constant7 : Constant  Value=decaytimes2  SampleTime=-1
  Constant8 : Constant  Value=conductancemaxima2  VectorParams1D=off  SampleTime=-1
  Discrete-Time Integrator : DiscreteIntegrator  gainval=1/stepsize  ExternalReset=sampled level  SampleTime=-1  ICPrevOutput=DiscIntNeverNeededParam  ICPrevScaledInput=DiscIntNeverNeededParam
  Discrete-Time Integrator1 : DiscreteIntegrator  gainval=1/stepsize  ExternalReset=sampled level  SampleTime=-1  ICPrevOutput=DiscIntNeverNeededParam  ICPrevScaledInput=DiscIntNeverNeededParam
  Floor1 : Rounding
  Floor2 : Rounding  Operator=round
  GC neuron : Subsystem
  Integrator1 : Integrator  ExternalReset=level hold
  Integrator2 : Integrator  ExternalReset=level hold
  MATLAB Function1 : MATLAB Function  TreatAsAtomicUnit=on
  MATLAB Function2 : MATLAB Function  TreatAsAtomicUnit=on
  Memory1 : Memory  InheritSampleTime=on
  Memory2 : Memory  InheritSampleTime=on
  Product2 : Product
  Product3 : Product
  To Workspace : ToWorkspace  VariableName=granulecell14_rasterplot  SampleTime=-1
  To Workspace1 : ToWorkspace  VariableName=granulecell14_v_scope  SampleTime=-1
  Uniform Random Number1 : UniformRandomNumber  Minimum=1  Maximum=noumberofevents  Seed=27  SampleTime=stepsize
  Uniform Random Number2 : UniformRandomNumber  Minimum=1  Maximum=noumberofevents  Seed=28  SampleTime=stepsize
  single exp EPSCs generator (recurrent synapse) : Subsystem
  single exp IPSCs generator (ihibitory synapse) : Subsystem
  GC output 14 : Outport
  tag scope: GC_14_current=global
  wires:
  GC neuron/1(v) -> To Workspace1/1
  GC neuron/2(output) -> To Workspace/1, GC output 14/1
  Constant7/1 -> MATLAB Function2/2(decaytimes2)
  Constant8/1 -> MATLAB Function2/3(conductancemaxima2)
  Discrete-Time Integrator1/1 -> MATLAB Function2/1(eventnoumber)
  Floor2/1 -> Product3/2
  Discrete-Time Integrator/1 -> MATLAB Function1/1(eventnoumber)
  MATLAB Function2/1(decaytime) -> single exp IPSCs generator (ihibitory synapse)/2(decay time constant)
  Product2/1 -> Discrete-Time Integrator/1
  Integrator2/1 -> single exp IPSCs generator (ihibitory synapse)/1(event time)
  Add/1 -> [GC_14_current], GC neuron/1(postsynaptic current)
  Memory2/1 -> Product3/1, Discrete-Time Integrator1/2, Integrator2/2
  single exp IPSCs generator (ihibitory synapse)/1(postsynaptic current) -> Add/2
  MATLAB Function1/1(decaytime) -> single exp EPSCs generator (recurrent synapse)/2(decay time constant)
  MATLAB Function1/2(conductancemaximum) -> single exp EPSCs generator (recurrent synapse)/3(conductance maximum)
  Constant6/1 -> Integrator2/1
  Constant4/1 -> MATLAB Function1/2(decaytimes1)
  Constant5/1 -> MATLAB Function1/3(conductancemaxima1)
  Integrator1/1 -> single exp EPSCs generator (recurrent synapse)/1(event time)
  Product3/1 -> Discrete-Time Integrator1/1
  single exp EPSCs generator (recurrent synapse)/1(postsynaptic current) -> Add/1
  lateral inhibition input/1 -> Memory2/1
  Floor1/1 -> Product2/2
  MATLAB Function2/2(conductancemaximum) -> single exp IPSCs generator (ihibitory synapse)/3(conductance maximum)
  Memory1/1 -> Product2/1, Discrete-Time Integrator/2, Integrator1/2
  Uniform Random Number1/1 -> Floor1/1
  Constant3/1 -> Integrator1/1
  Uniform Random Number2/1 -> Floor2/1
  excitatory input/1 -> Memory1/1

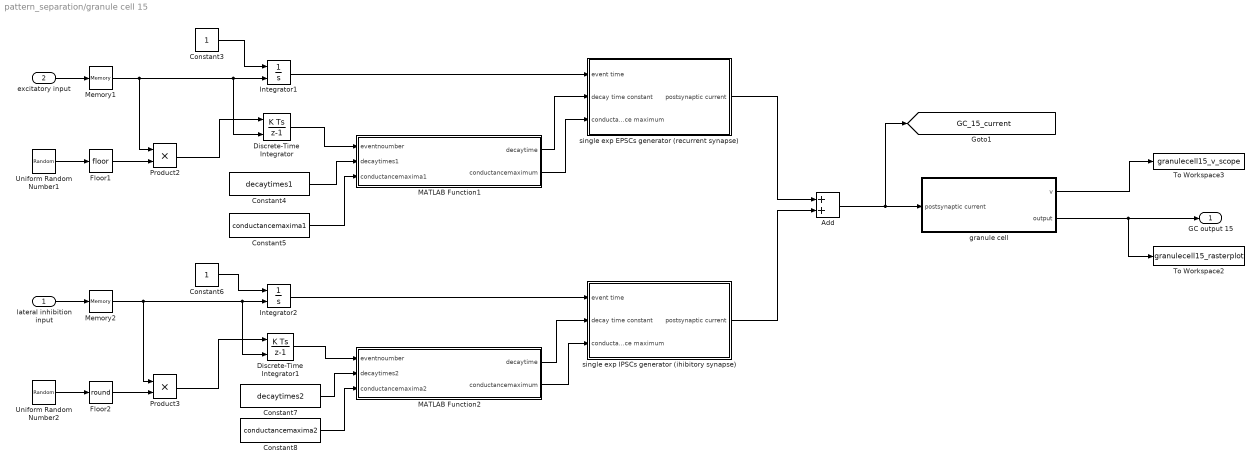
== system pattern_separation/granule cell 15 ==
  lateral inhibition input : Inport
  excitatory input : Inport  Port=2
  Add : Sum
  Constant3 : Constant  SampleTime=-1
  Constant4 : Constant  Value=decaytimes1  SampleTime=-1
  Constant5 : Constant  Value=conductancemaxima1  SampleTime=-1
  Constant6 : Constant  SampleTime=-1
  Constant7 : Constant  Value=decaytimes2  SampleTime=-1
  Constant8 : Constant  Value=conductancemaxima2  SampleTime=-1
  Discrete-Time Integrator : DiscreteIntegrator  gainval=1/stepsize  ExternalReset=sampled level  SampleTime=-1  ICPrevOutput=DiscIntNeverNeededParam  ICPrevScaledInput=DiscIntNeverNeededParam
  Discrete-Time Integrator1 : DiscreteIntegrator  gainval=1/stepsize  ExternalReset=sampled level  SampleTime=-1  ICPrevOutput=DiscIntNeverNeededParam  ICPrevScaledInput=DiscIntNeverNeededParam
  Floor1 : Rounding
  Floor2 : Rounding  Operator=round
  Integrator1 : Integrator  ExternalReset=level hold
  Integrator2 : Integrator  ExternalReset=level hold
  MATLAB Function1 : MATLAB Function  TreatAsAtomicUnit=on
  MATLAB Function2 : MATLAB Function  TreatAsAtomicUnit=on
  Memory1 : Memory  InheritSampleTime=on
  Memory2 : Memory  InheritSampleTime=on
  Product2 : Product
  Product3 : Product
  To Workspace2 : ToWorkspace  VariableName=granulecell15_rasterplot  SampleTime=-1
  To Workspace3 : ToWorkspace  VariableName=granulecell15_v_scope  SampleTime=-1
  Uniform Random Number1 : UniformRandomNumber  Minimum=1  Maximum=noumberofevents  Seed=29  SampleTime=stepsize
  Uniform Random Number2 : UniformRandomNumber  Minimum=1  Maximum=noumberofevents  Seed=30  SampleTime=stepsize
  granule cell : Subsystem
  single exp EPSCs generator (recurrent synapse) : Subsystem
  single exp IPSCs generator (ihibitory synapse) : Subsystem
  GC output 15 : Outport
  tag scope: GC_15_current=global
  wires:
  Discrete-Time Integrator/1 -> MATLAB Function1/1(eventnoumber)
  Memory1/1 -> Product2/1, Discrete-Time Integrator/2, Integrator1/2
  granule cell/2(output) -> GC output 15/1, To Workspace2/1
  MATLAB Function2/2(conductancemaximum) -> single exp IPSCs generator (ihibitory synapse)/3(conductance maximum)
  lateral inhibition input/1 -> Memory2/1
  Uniform Random Number1/1 -> Floor1/1
  Uniform Random Number2/1 -> Floor2/1
  excitatory input/1 -> Memory1/1
  single exp EPSCs generator (recurrent synapse)/1(postsynaptic current) -> Add/1
  Product3/1 -> Discrete-Time Integrator1/1
  Floor1/1 -> Product2/2
  Constant3/1 -> Integrator1/1
  single exp IPSCs generator (ihibitory synapse)/1(postsynaptic current) -> Add/2
  Product2/1 -> Discrete-Time Integrator/1
  granule cell/1(v) -> To Workspace3/1
  MATLAB Function1/1(decaytime) -> single exp EPSCs generator (recurrent synapse)/2(decay time constant)
  MATLAB Function2/1(decaytime) -> single exp IPSCs generator (ihibitory synapse)/2(decay time constant)
  Add/1 -> [GC_15_current], granule cell/1(postsynaptic current)
  Integrator1/1 -> single exp EPSCs generator (recurrent synapse)/1(event time)
  Constant5/1 -> MATLAB Function1/3(conductancemaxima1)
  Memory2/1 -> Product3/1, Discrete-Time Integrator1/2, Integrator2/2
  MATLAB Function1/2(conductancemaximum) -> single exp EPSCs generator (recurrent synapse)/3(conductance maximum)
  Constant6/1 -> Integrator2/1
  Constant4/1 -> MATLAB Function1/2(decaytimes1)
  Constant7/1 -> MATLAB Function2/2(decaytimes2)
  Constant8/1 -> MATLAB Function2/3(conductancemaxima2)
  Floor2/1 -> Product3/2
  Integrator2/1 -> single exp IPSCs generator (ihibitory synapse)/1(event time)
  Discrete-Time Integrator1/1 -> MATLAB Function2/1(eventnoumber)

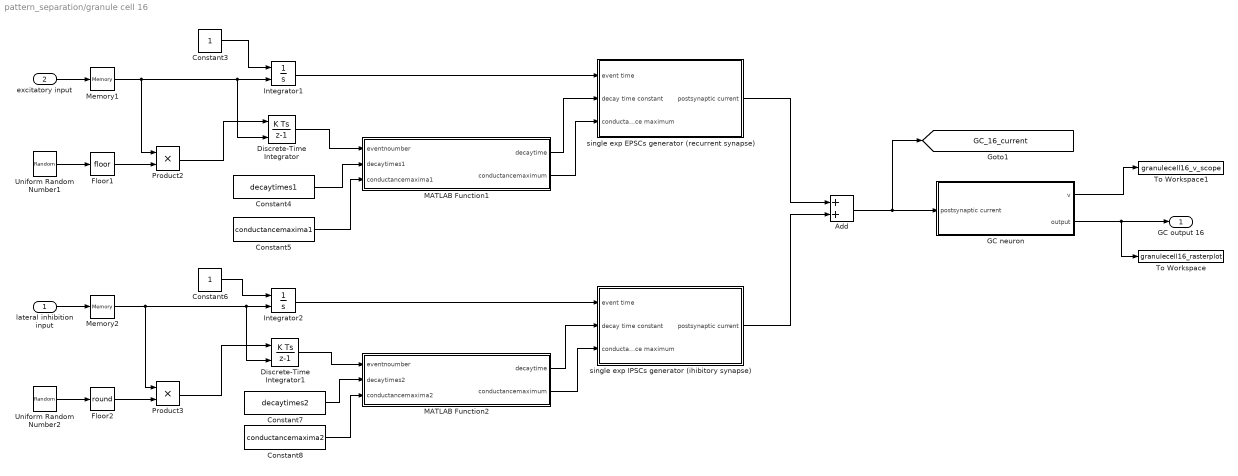
== system pattern_separation/granule cell 16 ==
  lateral inhibition input : Inport
  excitatory input : Inport  Port=2
  Add : Sum
  Constant3 : Constant  SampleTime=-1
  Constant4 : Constant  Value=decaytimes1  SampleTime=-1
  Constant5 : Constant  Value=conductancemaxima1  SampleTime=-1
  Constant6 : Constant  SampleTime=-1
  Constant7 : Constant  Value=decaytimes2  SampleTime=-1
  Constant8 : Constant  Value=conductancemaxima2  VectorParams1D=off  SampleTime=-1
  Discrete-Time Integrator : DiscreteIntegrator  gainval=1/stepsize  ExternalReset=sampled level  SampleTime=-1  ICPrevOutput=DiscIntNeverNeededParam  ICPrevScaledInput=DiscIntNeverNeededParam
  Discrete-Time Integrator1 : DiscreteIntegrator  gainval=1/stepsize  ExternalReset=sampled level  SampleTime=-1  ICPrevOutput=DiscIntNeverNeededParam  ICPrevScaledInput=DiscIntNeverNeededParam
  Floor1 : Rounding
  Floor2 : Rounding  Operator=round
  GC neuron : Subsystem
  Integrator1 : Integrator  ExternalReset=level hold
  Integrator2 : Integrator  ExternalReset=level hold
  MATLAB Function1 : MATLAB Function  TreatAsAtomicUnit=on
  MATLAB Function2 : MATLAB Function  TreatAsAtomicUnit=on
  Memory1 : Memory  InheritSampleTime=on
  Memory2 : Memory  InheritSampleTime=on
  Product2 : Product
  Product3 : Product
  To Workspace : ToWorkspace  VariableName=granulecell16_rasterplot  SampleTime=-1
  To Workspace1 : ToWorkspace  VariableName=granulecell16_v_scope  SampleTime=-1
  Uniform Random Number1 : UniformRandomNumber  Minimum=1  Maximum=noumberofevents  Seed=31  SampleTime=stepsize
  Uniform Random Number2 : UniformRandomNumber  Minimum=1  Maximum=noumberofevents  Seed=32  SampleTime=stepsize
  single exp EPSCs generator (recurrent synapse) : Subsystem
  single exp IPSCs generator (ihibitory synapse) : Subsystem
  GC output 16 : Outport
  tag scope: GC_16_current=global
  wires:
  GC neuron/1(v) -> To Workspace1/1
  GC neuron/2(output) -> To Workspace/1, GC output 16/1
  Constant7/1 -> MATLAB Function2/2(decaytimes2)
  Constant8/1 -> MATLAB Function2/3(conductancemaxima2)
  Discrete-Time Integrator1/1 -> MATLAB Function2/1(eventnoumber)
  Floor2/1 -> Product3/2
  Discrete-Time Integrator/1 -> MATLAB Function1/1(eventnoumber)
  MATLAB Function2/1(decaytime) -> single exp IPSCs generator (ihibitory synapse)/2(decay time constant)
  Product2/1 -> Discrete-Time Integrator/1
  Integrator2/1 -> single exp IPSCs generator (ihibitory synapse)/1(event time)
  Add/1 -> [GC_16_current], GC neuron/1(postsynaptic current)
  Memory2/1 -> Product3/1, Discrete-Time Integrator1/2, Integrator2/2
  single exp IPSCs generator (ihibitory synapse)/1(postsynaptic current) -> Add/2
  MATLAB Function1/1(decaytime) -> single exp EPSCs generator (recurrent synapse)/2(decay time constant)
  MATLAB Function1/2(conductancemaximum) -> single exp EPSCs generator (recurrent synapse)/3(conductance maximum)
  Constant6/1 -> Integrator2/1
  Constant4/1 -> MATLAB Function1/2(decaytimes1)
  Constant5/1 -> MATLAB Function1/3(conductancemaxima1)
  Integrator1/1 -> single exp EPSCs generator (recurrent synapse)/1(event time)
  Product3/1 -> Discrete-Time Integrator1/1
  single exp EPSCs generator (recurrent synapse)/1(postsynaptic current) -> Add/1
  lateral inhibition input/1 -> Memory2/1
  Floor1/1 -> Product2/2
  MATLAB Function2/2(conductancemaximum) -> single exp IPSCs generator (ihibitory synapse)/3(conductance maximum)
  Memory1/1 -> Product2/1, Discrete-Time Integrator/2, Integrator1/2
  Uniform Random Number1/1 -> Floor1/1
  Constant3/1 -> Integrator1/1
  Uniform Random Number2/1 -> Floor2/1
  excitatory input/1 -> Memory1/1
